simulink model "NLTRMS_2018a"  (R2018a)
settings: Solver=ode45  StartTime=0.0  StopTime=100  RelTol=1e-3  EnableMultiTasking=on
settings Model: Creator=morai
settings DataIOCC: LimitDataPoints=on
settings OptimizationCC: LifeSpan=inf
settings DebuggingCC: AllowSymbolicDim=off  SFUnexpectedBacktrackingDiag=warning  SFNoUnconditionalDefaultTransitionDiag=warning  SFExecutionAtInitializationDiag=none
settings ModelReferenceCC: PropagateSignalLabelsOutOfModel=off
settings CodeAppCC: StateflowObjectComments=on
settings GRTTargetCC: TargetLangStandard=C89/C90 (ANSI)
settings ConfigComp: CovMetricSettings=dw  CovSaveCumulativeToWorkspaceVar=on  CovSaveSingleToWorkspaceVar=on  CovExternalEMLEnable=off

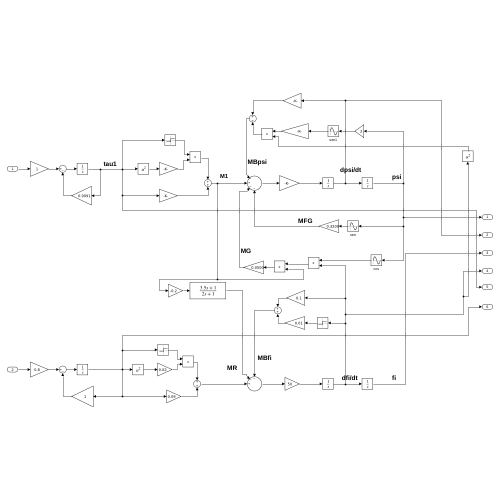
[thumbnail: Simulink's stored preview of the top-level diagram]
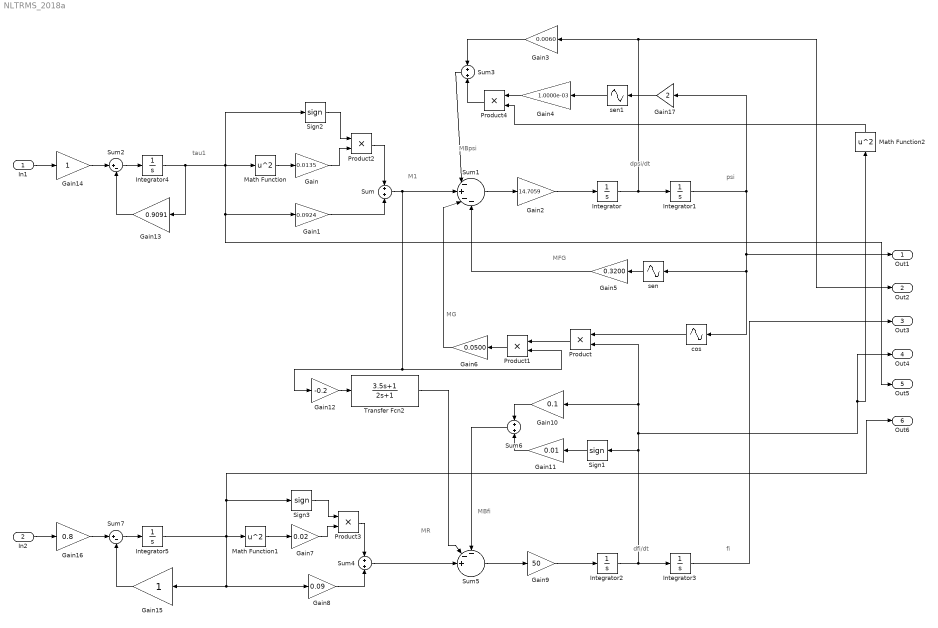
== system NLTRMS_2018a ==
  note: MR
  note: MBpsi
  note: MBfi
  note: tau1
  note: M1
  note: psi
  note: dfi/dt
  note: fi
  note: MG
  note: dpsi/dt
  note: MFG
  In1 : Inport
  In2 : Inport  Port=2
  Gain : Gain  Gain=0.0135
  Gain1 : Gain  Gain=0.0924
  Gain10 : Gain  Gain=0.1
  Gain11 : Gain  Gain=0.01
  Gain12 : Gain  Gain=-0.2
  Gain13 : Gain  Gain=0.9091
  Gain14 : Gain
  Gain15 : Gain
  Gain16 : Gain  Gain=0.8
  Gain17 : Gain  Gain=2
  Gain2 : Gain  Gain=14.7059
  Gain3 : Gain  Gain=0.0060
  Gain4 : Gain  Gain=1.0000e-03
  Gain5 : Gain  Gain=0.3200
  Gain6 : Gain  Gain=0.0500
  Gain7 : Gain  Gain=0.02
  Gain8 : Gain  Gain=0.09
  Gain9 : Gain  Gain=50
  Integrator{,1..5} (6 alike) : Integrator
  Math Function : Math  Operator=square  SaturateOnIntegerOverflow=on
  Math Function1 : Math  Operator=square  SaturateOnIntegerOverflow=on
  Math Function2 : Math  Operator=square  SaturateOnIntegerOverflow=on
  Product{,1..4} (5 alike) : Product
  Sign1 : Signum  ZeroCross=off
  Sign2 : Signum  ZeroCross=off
  Sign3 : Signum  ZeroCross=off
  Sum{,3..4,6} (4 alike) : Sum
  Sum1 : Sum  Inputs=|-+--
  Sum2 : Sum  Inputs=|+-
  Sum5 : Sum  Inputs=--+||
  Sum7 : Sum  Inputs=|+-
  Transfer Fcn2 : TransferFcn  Numerator=[3.5 1]  Denominator=[2 1]
  cos : Sin  TimeSource=Use external signal  Phase=pi/2  SampleTime=0
  sen : Sin  TimeSource=Use external signal  SampleTime=0
  sen1 : Sin  TimeSource=Use external signal  SampleTime=0
  Out1 : Outport  VectorParamsAs1DForOutWhenUnconnected=off
  Out2 : Outport  Port=2  VectorParamsAs1DForOutWhenUnconnected=off
  Out3 : Outport  Port=3  VectorParamsAs1DForOutWhenUnconnected=off
  Out4 : Outport  Port=4  VectorParamsAs1DForOutWhenUnconnected=off
  Out5 : Outport  Port=5  VectorParamsAs1DForOutWhenUnconnected=off
  Out6 : Outport  Port=6  VectorParamsAs1DForOutWhenUnconnected=off
  wires:
  Math Function2/1 -> Product4/2
  Product4/1 -> Sum3/2
  Product1/1 -> Gain6/1
  Transfer Fcn2/1 -> Sum5/2
  Gain6/1 -> Sum1/3
  Gain17/1 -> sen1/1
  Sum1/1 -> Gain2/1
  sen1/1 -> Gain4/1
  Math Function1/1 -> Gain7/1
  Gain4/1 -> Product4/1
  Gain7/1 -> Product3/2
  Sum4/1 -> Sum5/3
  Sum6/1 -> Sum5/1
  In1/1 -> Gain14/1
  In2/1 -> Gain16/1
  Gain12/1 -> Transfer Fcn2/1
  Integrator3/1 -> Out3/1
  Gain2/1 -> Integrator/1
  sen/1 -> Gain5/1
  Math Function/1 -> Gain/1
  Integrator1/1 -> cos/1, sen/1, Out1/1, Gain17/1
  Sign1/1 -> Gain11/1
  Gain14/1 -> Sum2/1
  Sum/1 -> Product1/2, Gain12/1, Sum1/2
  Gain9/1 -> Integrator2/1
  Sum5/1 -> Gain9/1
  Gain8/1 -> Sum4/2
  Product/1 -> Product1/1
  Integrator2/1 -> Product/2, Gain10/1, Out4/1, Math Function2/1, Sign1/1, Integrator3/1
  Gain10/1 -> Sum6/1
  Product2/1 -> Sum/1
  Gain15/1 -> Sum7/2
  Gain/1 -> Product2/2
  cos/1 -> Product/1
  Sum2/1 -> Integrator4/1
  Gain16/1 -> Sum7/1
  Gain5/1 -> Sum1/4
  Gain1/1 -> Sum/2
  Gain3/1 -> Sum3/1
  Sign3/1 -> Product3/1
  Integrator5/1 -> Math Function1/1, Sign3/1, Out6/1, Gain8/1, Gain15/1
  Sum3/1 -> Sum1/1
  Integrator4/1 -> Gain13/1, Sign2/1, Math Function/1, Out5/1, Gain1/1
  Sum7/1 -> Integrator5/1
  Product3/1 -> Sum4/1
  Integrator/1 -> Out2/1, Gain3/1, Integrator1/1
  Gain11/1 -> Sum6/2
  Gain13/1 -> Sum2/2
  Sign2/1 -> Product2/1
